simulink model "sampleModel2056"  (R2023a)
settings: Solver=VariableStepAuto  StartTime=0.0  StopTime=10.0  RelTol=1e-3
libraries: hdlsllib x4
settings Model: Creator=user1  LastModifiedBy=user1

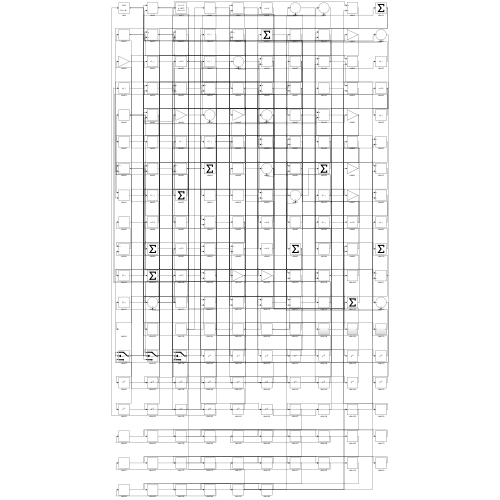
[thumbnail: Simulink's stored preview of the top-level diagram]
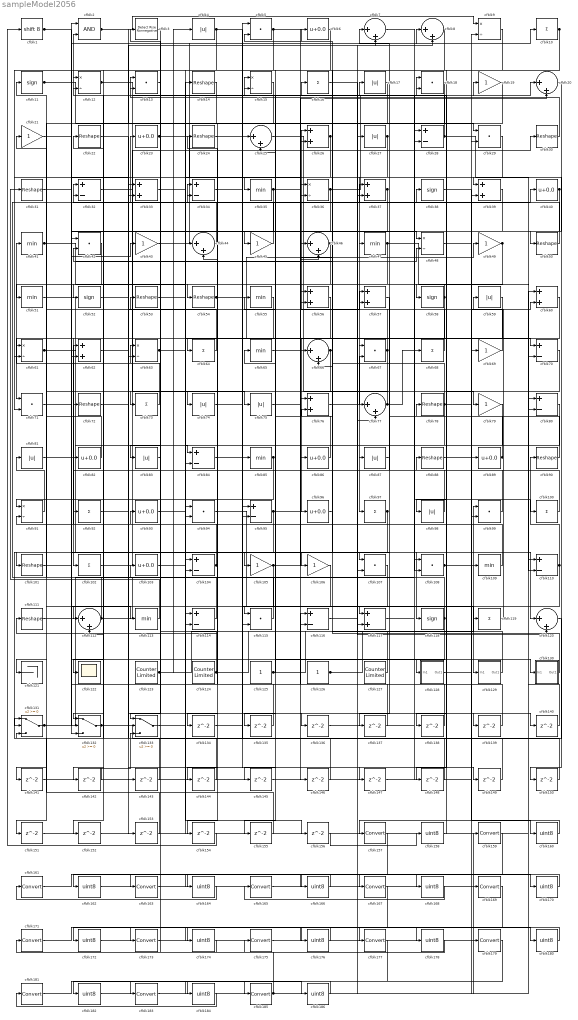
== system sampleModel2056 ==
  cfblk1 : ArithShift  BitShiftNumber=8
  cfblk{10,16,64,68,73,92,97,100,102,119} (10 alike) : Sum  Inputs=+
  cfblk{14,22,24,30..31,50,53..54,72,78,88,90,101,111} (14 alike) : Reshape
  cfblk{6,23,40,82,86,89,93,96,103} (9 alike) : Bias  Bias=0.0  SaturateOnIntegerOverflow=off
  cfblk{28,32,34,70,80,84,95,104,110,114,116} (11 alike) : Sum  Inputs=+-
  cfblk{19,21,43,45,49,69,79,105..106} (9 alike) : Gain
  cfblk{5,13,18,29,42,67,71,94,99,107..108,115} (12 alike) : DotProduct  OutDataTypeStr=Inherit: Inherit via internal rule
  cfblk{35,41,47,51,55,65,85,109,113} (9 alike) : MinMax
  cfblk{11,38,52,58,118} (5 alike) : Signum
  cfblk{7..8,20,25,44,46,66,77,112,120} (10 alike) : Sum  Inputs=|++
  cfblk{26,33,37,39,56..57,60,62,76,117} (10 alike) : Sum
  cfblk{9,12,15,36,48,61,63,91} (8 alike) : Product  Inputs=*/  RndMeth=Zero  SaturateOnIntegerOverflow=on
  cfblk121 : Terminator
  cfblk122 : Scope
  cfblk123 : hdlsllib/Sources/Counter Limited  uplimit=7  tsamp=-1
  cfblk124 : hdlsllib/Sources/Counter Limited  uplimit=7  tsamp=-1
  cfblk125 : Constant  SampleTime=-1
  cfblk126 : Constant  SampleTime=-1
  cfblk127 : hdlsllib/Sources/Counter Limited  uplimit=7  tsamp=-1
  cfblk128 : Subsystem
      settings: LibrarySourceBlock=|
      | hdlsllib/Ports &
      | Subsystems/Subsystem
  cfblk129 : Subsystem
      settings: LibrarySourceBlock=|
      | hdlsllib/Ports &
      | Subsystems/Subsystem
  cfblk130 : Subsystem
      settings: LibrarySourceBlock=|
      | hdlsllib/Ports &
      | Subsystems/Subsystem
  cfblk131 : Switch  SaturateOnIntegerOverflow=off  InputSameDT=off
  cfblk132 : Switch  SaturateOnIntegerOverflow=off  InputSameDT=off
  cfblk133 : Switch  SaturateOnIntegerOverflow=off  InputSameDT=off
  cfblk{134..156} (23 alike) : Delay  SampleTime=1
  cfblk{157,159,161,163,165,167,169,171,173,175,177,179,181,183,185} (15 alike) : DataTypeConversion  SaturateOnIntegerOverflow=off  RndMeth=Floor
  cfblk{158,160,162,164,166,168,170,172,174,176,178,180,182,184,186} (15 alike) : DataTypeConversion  OutDataTypeStr=uint8  SaturateOnIntegerOverflow=off  RndMeth=Floor
  cfblk{4,17,27,59,74..75,81,83,87,98} (10 alike) : Abs  SaturateOnIntegerOverflow=off
  cfblk2 : Logic  AllPortsSameDT=off  OutDataTypeStr=boolean
  cfblk3 : hdlsllib/Logic and Bit Operations/Detect Rise Nonnegative  vinit=0  OutDataTypeStr=boolean
  wires:
  cfblk12/1 -> cfblk75/1, cfblk20/1
  cfblk125/1 -> cfblk15/1, cfblk69/1
  cfblk56/1 -> cfblk102/1
  cfblk73/1 -> cfblk41/1
  cfblk43/1 -> cfblk8/1
  cfblk51/1 -> cfblk84/1
  cfblk8/1 -> cfblk106/1
  cfblk2/1 -> cfblk9/1, cfblk29/1
  cfblk47/1 -> cfblk80/2, cfblk134/1
  cfblk114/1 -> cfblk32/1
  cfblk61/1 -> cfblk118/1, cfblk104/2
  cfblk102/1 -> cfblk26/1
  cfblk46/1 -> cfblk54/1, cfblk66/2
  cfblk104/1 -> cfblk111/1, cfblk21/1
  cfblk113/1 -> cfblk31/1
  cfblk67/1 -> cfblk6/1, cfblk107/2
  cfblk123/1 -> cfblk99/1, cfblk4/1
  cfblk119/1 -> cfblk78/1
  cfblk50/1 -> cfblk22/1
  cfblk30/1 -> cfblk13/1
  cfblk132/1 -> cfblk39/1, cfblk57/2
  cfblk133/1 -> cfblk44/1
  cfblk27/1 -> cfblk97/1, cfblk122/1, cfblk37/2
  cfblk58/1 -> cfblk51/1, cfblk117/2, cfblk112/2
  cfblk44/1 -> cfblk34/1
  cfblk60/1 -> cfblk87/1
  cfblk25/1 -> cfblk79/1
  cfblk59/1 -> cfblk96/1
  cfblk111/1 -> cfblk103/1
  cfblk80/1 -> cfblk84/2
  cfblk131/1 -> cfblk28/1, cfblk37/1
  cfblk77/1 -> cfblk76/1, cfblk68/1
  cfblk98/1 -> cfblk62/1
  cfblk42/1 -> cfblk52/1
  cfblk81/1 -> cfblk120/1
  cfblk103/1 -> cfblk14/1
  cfblk71/1 -> cfblk42/1
  cfblk99/1 -> cfblk17/1
  cfblk101/1 -> cfblk43/1
  cfblk45/1 -> cfblk23/1
  cfblk10/1 -> cfblk115/1, cfblk58/1
  cfblk28/1 -> cfblk2/2, cfblk110/1
  cfblk29/1 -> cfblk73/1
  cfblk109/1 -> cfblk82/1
  cfblk79/1 -> cfblk115/2
  cfblk17/1 -> cfblk64/1
  cfblk33/1 -> cfblk30/1
  cfblk55/1 -> cfblk71/1
  cfblk90/1 -> cfblk16/1
  cfblk91/1 -> cfblk81/1
  cfblk5/1 -> cfblk117/1, cfblk152/1
  cfblk6/1 -> cfblk71/2
  cfblk94/1 -> cfblk129/1(In1)
  cfblk124/1 -> cfblk63/1, cfblk77/2
  cfblk53/1 -> cfblk67/1
  cfblk3/1 -> cfblk133/1
  cfblk105/1 -> cfblk40/1, cfblk132/3, cfblk65/1
  cfblk66/1 -> cfblk86/1, cfblk141/1, cfblk142/1
  cfblk82/1 -> cfblk61/1
  cfblk48/1 -> cfblk89/1
  cfblk68/1 -> cfblk26/2
  cfblk36/1 -> cfblk18/1, cfblk72/1
  cfblk96/1 -> cfblk46/1
  cfblk24/1 -> cfblk47/1
  cfblk118/1 -> cfblk53/1, cfblk55/1, cfblk145/1
  cfblk13/1 -> cfblk83/1
  cfblk130/1(Out1) -> cfblk56/1
  cfblk26/1 -> cfblk61/2, cfblk112/1
  cfblk129/1(Out1) -> cfblk36/1
  cfblk100/1 -> cfblk12/1
  cfblk76/1 -> cfblk67/2
  cfblk54/1 -> cfblk70/1, cfblk49/1
  cfblk21/1 -> cfblk48/1
  cfblk63/1 -> cfblk57/1, cfblk136/1
  cfblk9/1 -> cfblk25/2
  cfblk49/1 -> cfblk98/1, cfblk74/1
  cfblk116/1 -> cfblk27/1
  cfblk23/1 -> cfblk66/1, cfblk35/1
  cfblk95/1 -> cfblk131/2, cfblk20/2
  cfblk87/1 -> cfblk7/1
  cfblk128/1(Out1) -> cfblk109/1
  cfblk86/1 -> cfblk15/2
  cfblk37/1 -> cfblk62/2, cfblk45/1
  cfblk83/1 -> cfblk3/1
  cfblk117/1 -> cfblk19/1
  cfblk15/1 -> cfblk132/1
  cfblk32/1 -> cfblk108/2
  cfblk41/1 -> cfblk104/1, cfblk48/2, cfblk113/1
  cfblk7/1 -> cfblk99/2
  cfblk112/1 -> cfblk94/1, cfblk5/1, cfblk91/2
  cfblk64/1 -> cfblk11/1
  cfblk4/1 -> cfblk94/2, cfblk110/2
  cfblk19/1 -> cfblk92/1
  cfblk108/1 -> cfblk60/2, cfblk38/1
  cfblk20/1 -> cfblk50/1
  cfblk34/1 -> cfblk85/1
  cfblk16/1 -> cfblk120/2
  cfblk115/1 -> cfblk24/1
  cfblk11/1 -> cfblk95/2, cfblk46/2
  cfblk110/1 -> cfblk90/1, cfblk155/1
  cfblk14/1 -> cfblk132/2
  cfblk35/1 -> cfblk56/2, cfblk154/1
  cfblk97/1 -> cfblk105/1, cfblk121/1
  cfblk69/1 -> cfblk36/2
  cfblk78/1 -> cfblk39/2, cfblk107/1, cfblk5/2, cfblk42/2
  cfblk85/1 -> cfblk114/2, cfblk101/1
  cfblk31/1 -> cfblk10/1
  cfblk126/1 -> cfblk130/1(In1), cfblk119/1
  cfblk127/1 -> cfblk76/2
  cfblk40/1 -> cfblk63/2, cfblk135/1
  cfblk18/1 -> cfblk91/1
  cfblk84/1 -> cfblk116/2
  cfblk1/1 -> cfblk33/2, cfblk128/1(In1)
  cfblk38/1 -> cfblk100/1
  cfblk89/1 -> cfblk12/2, cfblk59/1
  cfblk72/1 -> cfblk8/2
  cfblk134/1 -> cfblk25/1
  cfblk135/1 -> cfblk34/2
  cfblk136/1 -> cfblk108/1
  cfblk57/1 -> cfblk137/1
  cfblk137/1 -> cfblk116/1
  cfblk39/1 -> cfblk138/1
  cfblk138/1 -> cfblk44/2
  cfblk65/1 -> cfblk139/1
  cfblk139/1 -> cfblk2/1
  cfblk62/1 -> cfblk140/1
  cfblk140/1 -> cfblk60/1
  cfblk141/1 -> cfblk9/2
  cfblk142/1 -> cfblk133/3
  cfblk52/1 -> cfblk143/1
  cfblk143/1 -> cfblk33/1
  cfblk107/1 -> cfblk144/1
  cfblk144/1 -> cfblk32/2
  cfblk145/1 -> cfblk7/2
  cfblk75/1 -> cfblk146/1
  cfblk146/1 -> cfblk133/2
  cfblk22/1 -> cfblk147/1
  cfblk147/1 -> cfblk28/2
  cfblk70/1 -> cfblk148/1
  cfblk148/1 -> cfblk131/1
  cfblk74/1 -> cfblk149/1
  cfblk149/1 -> cfblk95/1
  cfblk120/1 -> cfblk150/1
  cfblk150/1 -> cfblk18/2
  cfblk106/1 -> cfblk151/1
  cfblk151/1 -> cfblk114/1
  cfblk152/1 -> cfblk80/1
  cfblk92/1 -> cfblk153/1
  cfblk153/1 -> cfblk131/3
  cfblk154/1 -> cfblk1/1
  cfblk155/1 -> cfblk13/2
  cfblk93/1 -> cfblk156/1
  cfblk156/1 -> cfblk158/1
  cfblk158/1 -> cfblk88/1
  cfblk88/1 -> cfblk160/1
  cfblk160/1 -> cfblk157/1
  cfblk157/1 -> cfblk162/1
  cfblk162/1 -> cfblk159/1
  cfblk159/1 -> cfblk164/1
  cfblk164/1 -> cfblk161/1
  cfblk161/1 -> cfblk166/1
  cfblk166/1 -> cfblk163/1
  cfblk163/1 -> cfblk168/1
  cfblk168/1 -> cfblk165/1
  cfblk165/1 -> cfblk170/1
  cfblk170/1 -> cfblk167/1
  cfblk167/1 -> cfblk172/1
  cfblk172/1 -> cfblk169/1
  cfblk169/1 -> cfblk174/1
  cfblk174/1 -> cfblk171/1
  cfblk171/1 -> cfblk176/1
  cfblk176/1 -> cfblk173/1
  cfblk173/1 -> cfblk178/1
  cfblk178/1 -> cfblk175/1
  cfblk175/1 -> cfblk180/1
  cfblk180/1 -> cfblk177/1
  cfblk177/1 -> cfblk182/1
  cfblk182/1 -> cfblk179/1
  cfblk183/1 -> cfblk185/1
  cfblk179/1 -> cfblk184/1
  cfblk184/1 -> cfblk181/1
  cfblk185/1 -> cfblk29/2, cfblk77/1, cfblk70/2, cfblk93/1
  cfblk181/1 -> cfblk186/1
  cfblk186/1 -> cfblk183/1

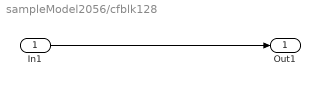
== system sampleModel2056/cfblk128 ==
  In1 : Inport
  Out1 : Outport
  wires:
  In1/1 -> Out1/1

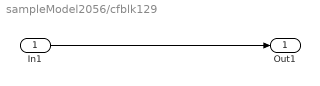
== system sampleModel2056/cfblk129 ==
  In1 : Inport
  Out1 : Outport
  wires:
  In1/1 -> Out1/1

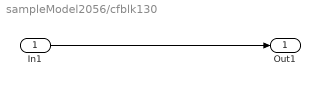
== system sampleModel2056/cfblk130 ==
  In1 : Inport
  Out1 : Outport
  wires:
  In1/1 -> Out1/1
